simulink model "Problem3"  (R2020b)
settings: Solver=VariableStepAuto  StartTime=0.0  StopTime=1  RelTol=1e-3
settings Model: Creator=ASUS  LastModifiedBy=ASUS

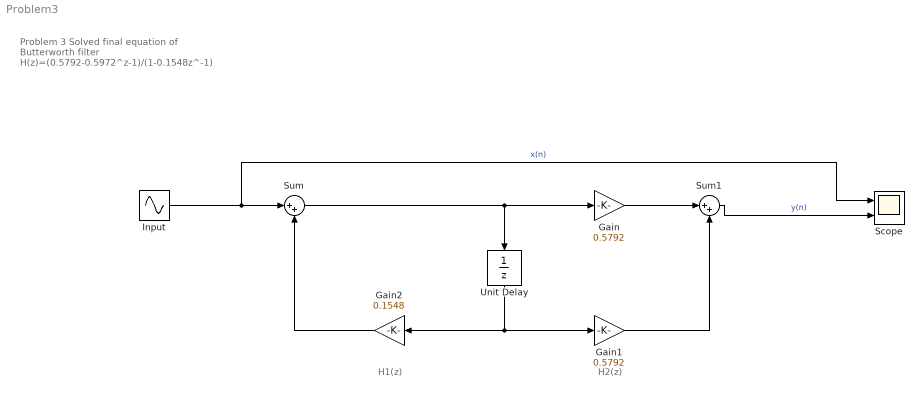
== system Problem3 ==
  note: H1(z)
  note: H2(z)
  note: Problem 3
      | Solved final equation of Butterworth filter
      | H(z)=(0.5792-0.5972^z-1)/(1-0.1548z^-1)
  Gain : Gain  Gain=0.5792
  Gain1 : Gain  Gain=0.5792
  Gain2 : Gain  Gain=0.1548
  Input : Sin  Frequency=5000  SampleTime=0
  Scope : Scope  NumInputPorts=2
  Sum : Sum  Inputs=|++
  Sum1 : Sum  Inputs=|++
  Unit Delay : UnitDelay  SampleTime=-1  HasFrameUpgradeWarning=on
  wires:
  Unit Delay/1 -> Gain2/1, Gain1/1
  Sum/1 -> Gain/1, Unit Delay/1
  Gain/1 -> Sum1/1
  Gain1/1 -> Sum1/2
  Gain2/1 -> Sum/2
  Sum1/1 -> Scope/2  "y(n)"
  Input/1 -> Scope/1, Sum/1  "x(n)"
